simulink model "test_ruido"  (R2020a)
settings: Solver=VariableStepAuto  StartTime=0.0  StopTime=20  MaxStep=1/fs  RelTol=1e-3
undefined symbols (not defined in the file): fs, NSD_mems
libraries: simulink x3, dspsrcs4 x1
settings Model: Creator=Noxi-PC  LastModifiedBy=Noxi-PC

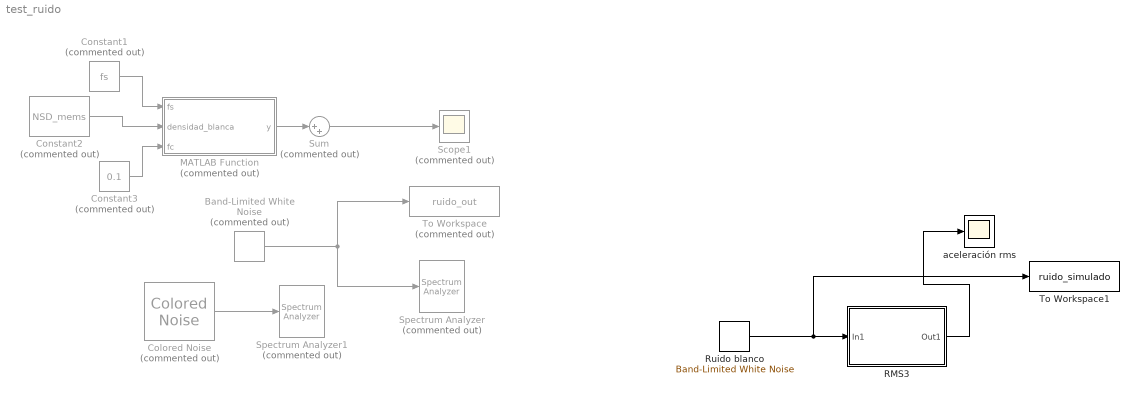
== system test_ruido ==
  Band-Limited White Noise : simulink/Sources/Band-Limited White Noise  Commented=on  Cov=NoisePower_mems  Ts=1/fs  seed=[23341]
  Colored Noise : dspsrcs4/Colored Noise  Commented=on  Color=pink  InverseFrequencyPower=1  BoundedOutput=on  NumChannels=1  OutputDataType=double  SamplesPerFrame=1  SampleTime=1/fs  RandomStream=mt19937ar with seed  Seed=67  SimulateUsing=Interpreted execution
      settings: SourceProductBaseCode=DS
  Constant1 : Constant  Commented=on  Value=fs
  Constant2 : Constant  Commented=on  Value=NSD_mems
  Constant3 : Constant  Commented=on  Value=0.1
  MATLAB Function : MATLAB Function  Commented=on  TreatAsAtomicUnit=on
  RMS3 : Subsystem
  Ruido blanco : simulink/Sources/Band-Limited White Noise  Cov=(30*9.81*10^(-6))^2  Ts=1/(fs)  seed=[2674]
  Scope1 : Scope  Commented=on
  Spectrum Analyzer : SpectrumAnalyzer  Commented=on
  Spectrum Analyzer1 : SpectrumAnalyzer  Commented=on
  Sum : Sum  Commented=on  Inputs=|++
  To Workspace : ToWorkspace  Commented=on  VariableName=ruido_out  SampleTime=-1
      settings: Save2DSignal=2-D array (concatenate along first dimension)
  To Workspace1 : ToWorkspace  VariableName=ruido_simulado  SaveFormat=Structure With Time  SampleTime=-1
  aceleración rms : Scope
  wires:
  Constant3/1 -> MATLAB Function/3(fc)
  Constant1/1 -> MATLAB Function/1(fs)
  Constant2/1 -> MATLAB Function/2(densidad_blanca)
  MATLAB Function/1(y) -> Sum/1
  Sum/1 -> Scope1/1
  Band-Limited White Noise/1 -> To Workspace/1, Spectrum Analyzer/1
  Colored Noise/1 -> Spectrum Analyzer1/1
  RMS3/1(Out1) -> aceleración rms/1
  Ruido blanco/1 -> To Workspace1/1, RMS3/1(In1)

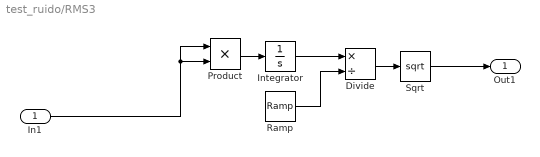
== system test_ruido/RMS3 ==
  In1 : Inport
  Divide : Product  Inputs=*/
  Integrator : Integrator
  Product : Product
  Ramp : simulink/Sources/Ramp  slope=1  start=0  InitialOutput=0
  Sqrt : Sqrt  SaturateOnIntegerOverflow=on
  Out1 : Outport  VectorParamsAs1DForOutWhenUnconnected=off
  wires:
  Ramp/1 -> Divide/2
  Product/1 -> Integrator/1
  Integrator/1 -> Divide/1
  Sqrt/1 -> Out1/1
  Divide/1 -> Sqrt/1
  In1/1 -> Product/1, Product/2

== matlab function test_ruido/MATLAB Function ==
  data: fs input; y output; densidad_blanca input; fc input
function y = ruido_sensor(fs, densidad_blanca, fc)

% Persistent state
persistent b a z

if isempty(b)
    [b, a] = butter(1, fc/(fs/2));
    z = 0;  % Estado inicial del filtro
end

% Ruido blanco
ruido_blanco = densidad_blanca * randn * sqrt(fs);

% Ruido 1/f (drift)
[ruido_drift, z] = filter(b, a, randn, z);

% Señal total
y = ruido_blanco;
